simulink library "TestVelocityController_UL"  (R2020a)
settings: Solver=VariableStepAuto  StartTime=0.0  StopTime=10.0  RelTol=1e-3
undefined symbols (not defined in the file): t_stop_adj, UNCC
libraries: $bdroot x1
settings Model: Creator=John Jr  LastModifiedBy=John Jr
settings DataIOCC: ReturnWorkspaceOutputs=off
settings DebuggingCC: ArithmeticOperatorsInVariantConditions=warning
settings SFSimCC: CustomCodeUndefinedFunction=UseInterfaceOnly

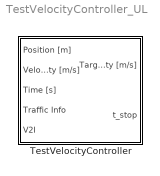
== system TestVelocityController_UL ==
  TestVelocityController : Subsystem
      mask Display:
      | patch([0 1 1 0], [0 0 1 1],[.8 1 1])
      | 
      | port_label('input',1,'Position','texmode','on')
      | port_label('input',2,'Velocity','texmode','on')
      | port_label('input',4,'Traffic','texmode','on')
      | port_label('input',3,'Time','texmode','on')
      | port_label('input',5,'V2I','texmode','on')
      | 
      | port_label('output',1,'V_{set}','texmode','on')
      | port_label('output',2,'t_{stop}','texmode','on')

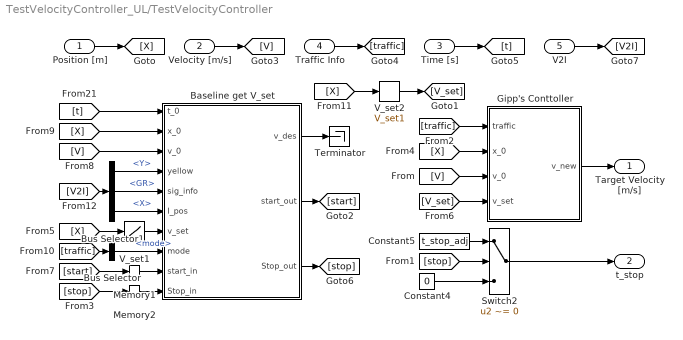
== system TestVelocityController_UL/TestVelocityController ==
  Position [m] : Inport
  Velocity [m/s] : Inport  Port=2
  Time [s] : Inport  Port=3
  Traffic Info : Inport  Port=4
  V2I : Inport  Port=5
  Baseline get V_set : MATLAB Function  TreatAsAtomicUnit=on
  Bus Selector : BusSelector  OutputSignals=mode
  Bus Selector1 : BusSelector  OutputSignals=Signal.Y,Signal.GR,Signal.X
  Constant4 : Constant  Value=0
  Constant5 : Constant  Value=t_stop_adj
  Gipp's Conttoller : MATLAB Function  TreatAsAtomicUnit=on
  Memory1 : Memory  InitialCondition=[0 0]
  Memory2 : Memory
  Switch2 : Switch  Criteria=u2 ~= 0
  Terminator : Terminator
  V_set1 : Lookup_n-D  NumberOfTableDimensions=1  BreakpointsForDimension1=UNCC.X_vec  Table=UNCC.V_lim  InterpMethod=Flat  ExtrapMethod=Clip  InputSameDT=on
  V_set2 : $bdroot/TestVelocityController/V_set1  NumberOfTableDimensions=1  DataSpecification=Table and breakpoints  BreakpointsSpecification=Explicit values  BreakpointsForDimension1=UNCC.X_vec  BreakpointsForDimension2=[10,22,31]  BreakpointsForDimension3=[1:3]  BreakpointsForDimension4=[1:3]  BreakpointsForDimension5=[1:3]  BreakpointsForDimension6=[1:3]  BreakpointsForDimension7=[1:3]  BreakpointsForDimension8=[1:3]  BreakpointsForDimension9=[1:3]  BreakpointsForDimension10=[1:3]  BreakpointsForDimension11=[1:3]  BreakpointsForDimension12=[1:3]  BreakpointsForDimension13=[1:3]  BreakpointsForDimension14=[1:3]  BreakpointsForDimension15=[1:3]  BreakpointsForDimension16=[1:3]  BreakpointsForDimension17=[1:3]  BreakpointsForDimension18=[1:3]  BreakpointsForDimension19=[1:3]  BreakpointsForDimension20=[1:3]  BreakpointsForDimension21=[1:3]  BreakpointsForDimension22=[1:3]  BreakpointsForDimension23=[1:3]  BreakpointsForDimension24=[1:3]  BreakpointsForDimension25=[1:3]  BreakpointsForDimension26=[1:3]  BreakpointsForDimension27=[1:3]  BreakpointsForDimension28=[1:3]  BreakpointsForDimension29=[1:3]  BreakpointsForDimension30=[1:3]  BreakpointsForDimension1FirstPoint=1  BreakpointsForDimension2FirstPoint=1  BreakpointsForDimension3FirstPoint=1  BreakpointsForDimension4FirstPoint=1  BreakpointsForDimension5FirstPoint=1  BreakpointsForDimension6FirstPoint=1  BreakpointsForDimension7FirstPoint=1  BreakpointsForDimension8FirstPoint=1  BreakpointsForDimension9FirstPoint=1  BreakpointsForDimension10FirstPoint=1  BreakpointsForDimension11FirstPoint=1  BreakpointsForDimension12FirstPoint=1  BreakpointsForDimension13FirstPoint=1  BreakpointsForDimension14FirstPoint=1  BreakpointsForDimension15FirstPoint=1  BreakpointsForDimension16FirstPoint=1  BreakpointsForDimension17FirstPoint=1  BreakpointsForDimension18FirstPoint=1  BreakpointsForDimension19FirstPoint=1  BreakpointsForDimension20FirstPoint=1  BreakpointsForDimension21FirstPoint=1  BreakpointsForDimension22FirstPoint=1  BreakpointsForDimension23FirstPoint=1  BreakpointsForDimension24FirstPoint=1  BreakpointsForDimension25FirstPoint=1  BreakpointsForDimension26FirstPoint=1  BreakpointsForDimension27FirstPoint=1  BreakpointsForDimension28FirstPoint=1  BreakpointsForDimension29FirstPoint=1  BreakpointsForDimension30FirstPoint=1  BreakpointsForDimension1Spacing=1  BreakpointsForDimension2Spacing=1  BreakpointsForDimension3Spacing=1  BreakpointsForDimension4Spacing=1  BreakpointsForDimension5Spacing=1  BreakpointsForDimension6Spacing=1  BreakpointsForDimension7Spacing=1  BreakpointsForDimension8Spacing=1  BreakpointsForDimension9Spacing=1  BreakpointsForDimension10Spacing=1  BreakpointsForDimension11Spacing=1  BreakpointsForDimension12Spacing=1  BreakpointsForDimension13Spacing=1  BreakpointsForDimension14Spacing=1  BreakpointsForDimension15Spacing=1  BreakpointsForDimension16Spacing=1  BreakpointsForDimension17Spacing=1  BreakpointsForDimension18Spacing=1  BreakpointsForDimension19Spacing=1  BreakpointsForDimension20Spacing=1  BreakpointsForDimension21Spacing=1  BreakpointsForDimension22Spacing=1  BreakpointsForDimension23Spacing=1  BreakpointsForDimension24Spacing=1  BreakpointsForDimension25Spacing=1  BreakpointsForDimension26Spacing=1  BreakpointsForDimension27Spacing=1  BreakpointsForDimension28Spacing=1  BreakpointsForDimension29Spacing=1  BreakpointsForDimension30Spacing=1  BreakpointsForDimension1Min=[]  BreakpointsForDimension2Min=[]  BreakpointsForDimension3Min=[]  BreakpointsForDimension4Min=[]  BreakpointsForDimension5Min=[]  BreakpointsForDimension6Min=[]  BreakpointsForDimension7Min=[]  BreakpointsForDimension8Min=[]  BreakpointsForDimension9Min=[]  BreakpointsForDimension10Min=[]  BreakpointsForDimension11Min=[]  BreakpointsForDimension12Min=[]  BreakpointsForDimension13Min=[]  BreakpointsForDimension14Min=[]  BreakpointsForDimension15Min=[]  BreakpointsForDimension16Min=[]  BreakpointsForDimension17Min=[]  BreakpointsForDimension18Min=[]  BreakpointsForDimension19Min=[]  BreakpointsForDimension20Min=[]  BreakpointsForDimension21Min=[]  BreakpointsForDimension22Min=[]  BreakpointsForDimension23Min=[]  BreakpointsForDimension24Min=[]  BreakpointsForDimension25Min=[]  BreakpointsForDimension26Min=[]  BreakpointsForDimension27Min=[]  BreakpointsForDimension28Min=[]  BreakpointsForDimension29Min=[]  BreakpointsForDimension30Min=[]  BreakpointsForDimension1Max=[]  BreakpointsForDimension2Max=[]  BreakpointsForDimension3Max=[]  BreakpointsForDimension4Max=[]  BreakpointsForDimension5Max=[]  BreakpointsForDimension6Max=[]  BreakpointsForDimension7Max=[]  BreakpointsForDimension8Max=[]  BreakpointsForDimension9Max=[]  BreakpointsForDimension10Max=[]  BreakpointsForDimension11Max=[]  BreakpointsForDimension12Max=[]  BreakpointsForDimension13Max=[]  BreakpointsForDimension14Max=[]  BreakpointsForDimension15Max=[]  BreakpointsForDimension16Max=[]  BreakpointsForDimension17Max=[]  BreakpointsForDimension18Max=[]  BreakpointsForDimension19Max=[]  BreakpointsForDimension20Max=[]  BreakpointsForDimension21Max=[]  BreakpointsForDimension22Max=[]  BreakpointsForDimension23Max=[]  BreakpointsForDimension24Max=[]  BreakpointsForDimension25Max=[]  BreakpointsForDimension26Max=[]  BreakpointsForDimension27Max=[]  BreakpointsForDimension28Max=[]  BreakpointsForDimension29Max=[]  BreakpointsForDimension30Max=[]  BreakpointsForDimension1DataTypeStr=Inherit: Same as corresponding input  BreakpointsForDimension2DataTypeStr=Inherit: Same as corresponding input  BreakpointsForDimension3DataTypeStr=Inherit: Same as corresponding input  BreakpointsForDimension4DataTypeStr=Inherit: Same as corresponding input  BreakpointsForDimension5DataTypeStr=Inherit: Same as corresponding input  BreakpointsForDimension6DataTypeStr=Inherit: Same as corresponding input  BreakpointsForDimension7DataTypeStr=Inherit: Same as corresponding input  BreakpointsForDimension8DataTypeStr=Inherit: Same as corresponding input  BreakpointsForDimension9DataTypeStr=Inherit: Same as corresponding input  BreakpointsForDimension10DataTypeStr=Inherit: Same as corresponding input  BreakpointsForDimension11DataTypeStr=Inherit: Same as corresponding input  BreakpointsForDimension12DataTypeStr=Inherit: Same as corresponding input  BreakpointsForDimension13DataTypeStr=Inherit: Same as corresponding input  BreakpointsForDimension14DataTypeStr=Inherit: Same as corresponding input  BreakpointsForDimension15DataTypeStr=Inherit: Same as corresponding input  BreakpointsForDimension16DataTypeStr=Inherit: Same as corresponding input  BreakpointsForDimension17DataTypeStr=Inherit: Same as corresponding input  BreakpointsForDimension18DataTypeStr=Inherit: Same as corresponding input  BreakpointsForDimension19DataTypeStr=Inherit: Same as corresponding input  BreakpointsForDimension20DataTypeStr=Inherit: Same as corresponding input  BreakpointsForDimension21DataTypeStr=Inherit: Same as corresponding input  BreakpointsForDimension22DataTypeStr=Inherit: Same as corresponding input  BreakpointsForDimension23DataTypeStr=Inherit: Same as corresponding input  BreakpointsForDimension24DataTypeStr=Inherit: Same as corresponding input  BreakpointsForDimension25DataTypeStr=Inherit: Same as corresponding input  BreakpointsForDimension26DataTypeStr=Inherit: Same as corresponding input  BreakpointsForDimension27DataTypeStr=Inherit: Same as corresponding input  BreakpointsForDimension28DataTypeStr=Inherit: Same as corresponding input  BreakpointsForDimension29DataTypeStr=Inherit: Same as corresponding input  BreakpointsForDimension30DataTypeStr=Inherit: Same as corresponding input  IndexSearchMethod=Binary search  BeginIndexSearchUsingPreviousIndexResult=off  UseOneInputPortForAllInputData=off  Table=UNCC.V_lim  TableMin=[]  TableMax=[]  TableDataTypeStr=Inherit: Same as output  IntermediateResultsDataTypeStr=Inherit: Same as output  InterpMethod=Flat  ExtrapMethod=Clip  DiagnosticForOutOfRangeInput=None  RemoveProtectionInput=off  UseLastTableValue=off  SampleTime=-1  InternalRulePriority=Precision  InputSameDT=on  OutMin=[]  OutMax=[]  SupportTunableTableSize=off  MaximumIndicesForEachDimension=[]
  Target Velocity [m/s] : Outport  VectorParamsAs1DForOutWhenUnconnected=off
  t_stop : Outport  Port=2  VectorParamsAs1DForOutWhenUnconnected=off
  wires:
  Bus Selector1/3 -> Baseline get V_set/6(I_pos)  "<X>"
  Bus Selector1/2 -> Baseline get V_set/5(sig_info)  "<GR>"
  Bus Selector1/1 -> Baseline get V_set/4(yellow)  "<Y>"
  [V2I] -> Bus Selector1/1
  Bus Selector/1 -> Baseline get V_set/8(mode)  "<mode>"
  [traffic] -> Bus Selector/1
  Position [m]/1 -> [X]
  [traffic] -> Gipp's Conttoller/1(traffic)
  [X] -> Gipp's Conttoller/2(x_0)
  Traffic Info/1 -> [traffic]
  Velocity [m/s]/1 -> [V]
  [V] -> Gipp's Conttoller/3(v_0)
  Time [s]/1 -> [t]
  [X] -> V_set1/1
  [t] -> Baseline get V_set/1(t_0)
  V_set1/1 -> Baseline get V_set/7(v_set)
  [X] -> Baseline get V_set/2(x_0)
  [V] -> Baseline get V_set/3(v_0)
  [V_set] -> Gipp's Conttoller/4(v_set)
  Constant4/1 -> Switch2/3
  Constant5/1 -> Switch2/1
  Switch2/1 -> t_stop/1
  Baseline get V_set/2(start_out) -> [start]
  Baseline get V_set/3(Stop_out) -> [stop]
  [stop] -> Switch2/2
  Memory1/1 -> Baseline get V_set/9(start_in)
  Memory2/1 -> Baseline get V_set/10(Stop_in)
  [stop] -> Memory2/1
  [start] -> Memory1/1
  Gipp's Conttoller/1(v_new) -> Target Velocity [m/s]/1
  [X] -> V_set2/1
  V_set2/1 -> [V_set]
  Baseline get V_set/1(v_des) -> Terminator/1
  V2I/1 -> [V2I]

== matlab function TestVelocityController_UL/TestVelocityController/Baseline get V_set ==
  data: t_0 input; v_des output size=1; start_out output size=[1 2]; x_0 input; v_0 input; yellow input; sig_info input; I_pos input; v_set input; mode input; start_in input size=2; Stop_in input size=1; Stop_out output size=1
function [v_des,start_out,Stop_out] = fcn(t_0,x_0,v_0,yellow,sig_info,I_pos,v_set,mode,start_in,Stop_in)

G = sig_info(:,:,2);                                    %   s - Intersection green phases 
Cs = sig_info(:,:,3);                                   %   s - Cycle start times 
window = 150;                                           %   m - Driver sight range
dt = .01;                                               %   s - Sample time
Idx1 = find(x_0-I_pos < 0,1,'first');                   %   Next upcoming intersection 
if isempty(Idx1)
    dx = 500;
else
    dx = I_pos(Idx1(1))-x_0;                            %   m - Distance to upcoming intersection 
end
if dx >= window
    Int_approach = 0;                                   %   No upcoming intersection 
else
    Int_approach = 1;                                   %   There is an upcoming intersection 
end
if Int_approach == 1
    Idx2 = find(Cs(Idx1(1),:) <= t_0,1,'last');         %   Current cycle # for upcoming intersection
    x_approach = v_0*yellow(Idx1(1));                            %   m - Distance to make yellow
    if t_0 < Cs(Idx1(1),Idx2(1))+G(Idx1(1),Idx2(1))-yellow(Idx1(1))
        light = 0;                                      %   Light is green
    elseif t_0 >= Cs(Idx1(1),Idx2(1))+G(Idx1(1),Idx2(1))-yellow(Idx1(1))...
            && t_0 < Cs(Idx1(1),Idx2(1))+G(Idx1(1),Idx2(1))
        light = 1;                                      %   Light is yellow
    else
        light = 2;                                      %   Light is red
    end
    if light == 0 && Stop_in == 1
        Stop_out = 0;
        start_in = [0 0];
    elseif (light == 1 && dx > x_approach) || light == 2 ...
            || (light == 1 && Stop_in == 1)
        Stop_out = 1;
        start_in = start_in';
    else
        Stop_out = 0;
        start_in = [0 0];
    end
else
    Stop_out = 0;
    start_in = [0 0];
end
if Stop_out == 1 && start_in(1) == 0
    start_in = [x_0,v_0];
end
if Stop_out == 1
    if mode == 1
        x_stop = linspace(start_in(1),I_pos(Idx1(1))-15,100);
    else
        x_stop = linspace(start_in(1),I_pos(Idx1(1))-5,100);
    end
    v_stop = linspace(start_in(2),0,100);
    v_des = interp1(x_stop,v_stop,x_0,'linear',0);
else
    v_des = v_set;
end
start_out = start_in;
end

== matlab function TestVelocityController_UL/TestVelocityController/Gipp's Conttoller ==
  data: traffic input size=6; v_new output; x_0 input; v_0 input; v_set input
function v_new  = fcn(traffic,x_0,v_0,v_set)

tau = 0.75;                 %   s - Driver reaction time
a_n = 2;                    %   m/s^2 - Maximum acceleration
b_n = -2*a_n;               %   m/s^2 - Maximum brake acceleration
b_hat = -2;                 %   m/s^2 - Estimated lead vehicle brake acceleration
t_n = 2;                    %   s - Safe following time

x_lead = traffic(1);        %   m - Lead vehicle poaition
v_lead = traffic(2);        %   m/s - Lead vehicle velocity
s_n = max(v_lead*t_n,5);    %   m - Safe following distance
v_0 = max(v_0,0);

if x_lead-x_0 <= 0          %   Condition to prevent negative radical
    x_lead = x_0;
    v_lead = v_0;
end

if traffic(4) == 0        %   In traffic?
    v_new = v_set;
else
    if (b_n^2*tau^2-b_n*(2*(x_lead-s_n-x_0)-v_0*tau-v_lead^2/b_hat)) > 0
        v_new = min(v_0+2.5*a_n*tau*(1-v_0/v_set)*sqrt(.025+v_0/v_set),...
            b_n*tau+sqrt(b_n^2*tau^2-b_n*(2*(x_lead-s_n-x_0)-v_0*tau-v_lead^2/b_hat)));
    else
        v_new = 0;
    end
    v_new = max(v_new,0);
end
